simulink model "traiettoria_corretta (3)"  (R2022b)
settings: Solver=FixedStepAuto  StartTime=0.0  StopTime=70  RelTol=1e-3  EnableMultiTasking=on
PreLoadFcn:
  | if ispc
  | SampleTime = 0.01
  | PID_x_P = 8
  | PID_x_I = 0.1
  | PID_x_D = 10
  | PID_x_N = 10
  | 
  | PID_y_P = 8
  | PID_y_I = 0.1
  | PID_y_D = 6
  | PID_y_N = 10
  | 
  | PID_z_P = 1.13
  | PID_z_I = 0.1
  | PID_z_D = 0.8
  | PID_z_N = 100
  | 
  | PID_yaw_P = 0.08024000000000001
  | PID_yaw_I = 0.005
  | PID_yaw_D = 0.075
  | PID_yaw_N = 100
  | 
  | elseif isunix
  | SampleTime = 0.004
  | PID_x_P = 1
  | PID_x_I = 0.01
  | PID_x_D = 4
  | PID_x_N = 1
  | 
  | PID_y_P = 1
  | PID_y_I = 0.01
  | PID_y_D = 4
  | PID_y_N = 1
  | 
  | PID_z_P = 1
  | PID_z_I = 0.01
  | PID_z_D = 0.8
  | PID_z_N = 50
  | 
  | PID_yaw_P = 0.08024000000000001
  | PID_yaw_I = 0.005
  | PID_yaw_D = 0.075
  | PID_yaw_N = 100
  | end
undefined symbols (not defined in the file): dev, Main, pwm_output0
libraries: px4uORBlib x7, slpidlib x6, simulink_extras x3, px4Sensorslib x2, sharedtransform x1, SignalEditorBlockLib x1, px4lib x1
CloseFcn:
  | clear PID_yaw*;
  | clear PID_x*;
  | clear PID_y*;
  | clear PID_z*;
  | clear SampleTime;
settings Model: SimulationMode=external  ExtModeTrigDuration=3001  Creator=The MathWorks, Inc.  LastModifiedBy=utente
settings SolverCC: AlgebraicLoopSolver=TrustRegion  PositivePriorityOrder=on  AutoInsertRateTranBlk=on  MaxZcPerStep=1
settings OptimizationCC: EnhancedBackFolding=on  PassReuseOutputArgsAs=Individual arguments  ZeroExternalMemoryAtStartup=off  ZeroInternalMemoryAtStartup=off  MaxStackSize=64  OptimizeBlockOrder=speed  DifferentSizesBufferReuse=on  OptimizationCustomize=off  EfficientTunableParamExpr=on
settings DebuggingCC: MultiTaskDSMMsg=none  ParameterTunabilityLossMsg=error  UnconnectedInputMsg=warning  UnconnectedOutputMsg=warning  UnconnectedLineMsg=warning  SFMachineParentedDataDiag=warning
settings HardwareCC: ProdBitPerPointer=32  ProdBitPerSizeT=32  ProdBitPerPtrDiffT=32  ProdLargestAtomicInteger=Long  ProdLargestAtomicFloat=Double  ProdWordSize=32  ProdLongLongMode=on  ProdHWDeviceType=ARM Compatible->ARM Cortex
settings ModelReferenceCC: EnableRefExpFcnMdlSchedulingChecks=on
settings SFSimCC: MATLABDynamicMemAlloc=off  SimTargetLang=C++
settings RTWCC: Description=Embedded Coder  SystemTargetFile=ert.tlc  HardwareBoard=PX4 Host Target  TemplateMakefile=ert_default_tmf  Toolchain=GNU Tools for PX4 Autopilots  PortableWordSizes=on  TargetLang=C++  DLArmComputeVersion=19.05
settings CodeAppCC: ForceParamTrailComments=on  IgnoreCustomStorageClasses=off  OperatorAnnotations=on  SimulinkDataObjDesc=on  SFDataObjDesc=on  InsertBlockDesc=on
settings ERTTargetCC: ExtMode=on  ExtModeTransport=2  ExtModeStaticAlloc=on  ExtModeMexFile=ext_xcp  ExtModeMexArgs='127.0.0.1' 1 17725  ExtModeIntrfLevel=Level2 - Open

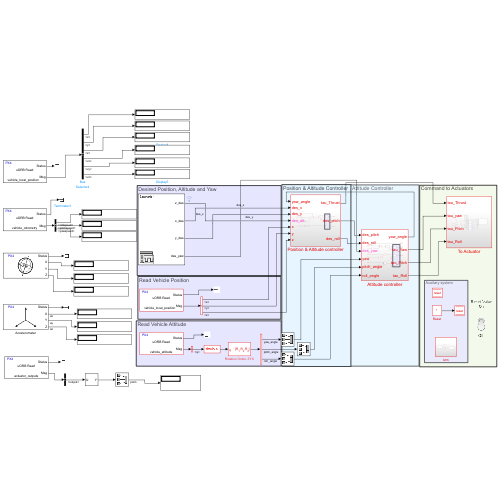
[thumbnail: Simulink's stored preview of the top-level diagram]
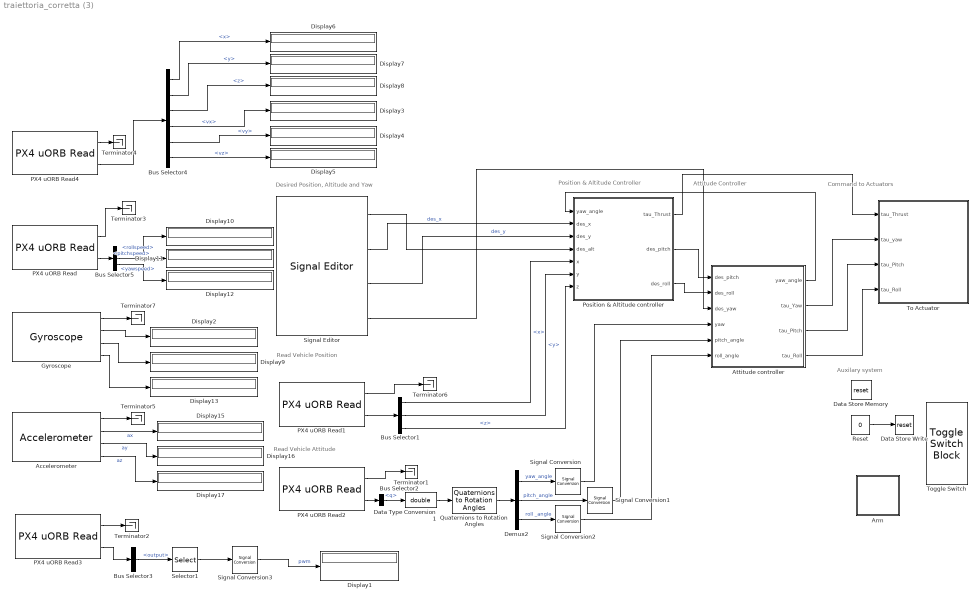
== system traiettoria_corretta (3) ==
  note: Read Vehicle Attitude
  note: Position & Altitude Controller
  note: Command to Actuators
  note: Auxilary system
  note: Attitude Controller
  note: Desired Position, Altitude and Yaw
  note: Read Vehicle Position
  Accelerometer : px4Sensorslib/Accelerometer  uorbTimeStamp=off  BlockingMode=off  BlockTimeout=1e-3  sampleTime=0.01
  Arm : Subsystem
  Attitude controller : Subsystem
  Bus Selector1 : BusSelector  OutputSignals=x,y,z
  Bus Selector2 : BusSelector  OutputSignals=q
  Bus Selector3 : BusSelector  OutputSignals=output
  Bus Selector4 : BusSelector  OutputSignals=x,y,z,vx,vy,vz
  Bus Selector5 : BusSelector  OutputSignals=rollspeed,pitchspeed,yawspeed
  Data Store Write : DataStoreWrite  DataStoreName=reset  IndexOptions=Index vector (dialog)  Indices=1  OutputSizes=1
  Data Store Memory : DataStoreMemory  DataStoreName=reset  ReadBeforeWriteMsg=warning  WriteAfterWriteMsg=warning  WriteAfterReadMsg=warning  ShowAdditionalParam=off  OutDataTypeStr=boolean
  Data Type Conversion1 : DataTypeConversion  OutDataTypeStr=double  SaturateOnIntegerOverflow=off  RndMeth=Floor
  Demux2 : Demux  Outputs=3
  Display{1..13,15..17} (16 alike) : Display
  Gyroscope : px4Sensorslib/Gyroscope  uorbTimeStamp=off  BlockingMode=off  BlockTimeout=1e-3  sampleTime=1/250
  PX4 uORB Read : px4uORBlib/PX4 uORB Read  uORBTopic=vehicle_odometry  selectInstance=vehicle_odometry  SampleTime=0.01  BlockingMode=off  BlockTimeout=1e-3
  PX4 uORB Read1 : px4uORBlib/PX4 uORB Read  uORBTopic=vehicle_local_position  selectInstance=vehicle_local_position_groundtruth  SampleTime=0.01  BlockingMode=off  BlockTimeout=1e-3
  PX4 uORB Read2 : px4uORBlib/PX4 uORB Read  uORBTopic=vehicle_attitude  selectInstance=vehicle_attitude_groundtruth  SampleTime=0.01  BlockingMode=off  BlockTimeout=1e-3
  PX4 uORB Read3 : px4uORBlib/PX4 uORB Read  uORBTopic=actuator_outputs  selectInstance=actuator_outputs  SampleTime=0.01  BlockingMode=off  BlockTimeout=1e-3
  PX4 uORB Read4 : px4uORBlib/PX4 uORB Read  uORBTopic=vehicle_local_position  selectInstance=vehicle_local_position_groundtruth  SampleTime=0.01  BlockingMode=off  BlockTimeout=1e-3
  Position & Altitude controller : Subsystem
  Quaternions to Rotation Angles : sharedtransform/Quaternions to Rotation Angles  rotationOrder=ZYX  aMode=aMode
  Reset : Constant  Value=0  OutDataTypeStr=boolean  SampleTime=-1
      settings: OpenFcn=|
      | if strcmp('0',get_param(gcb, 'Value'))                        set_param(gcb, 'Value', '1');
      | else
      |             set_param(gcb, 'Value', '0');
      | end
  Selector1 : Selector  InputPortWidth=16  IndexOptions=Index vector (dialog)  Indices=[1 2]  OutputSizes=1
  Signal Conversion{,1..3} (4 alike) : SignalConversion  OverrideOpt=off
  Signal Editor : SignalEditorBlockLib/Signal Editor  FileName=traiettoria_signal.mat  ActiveScenario=Scenario1  ActiveSignal=des_yaw  IsBus=off  OutputBusObjectStr=Bus: BusObject  SampleTime=0.01  Interpolate=off  ZeroCross=off  OutputAfterFinalValue=Setting to zero  Unit=inherit  PreserveSignalName=on
  Terminator{1..7} (7 alike) : Terminator
  To Actuator : Subsystem
  Toggle Switch : ToggleSwitchBlock
      settings: Values={{'Off', 'On'}, [0 1]}
  wires:
  Signal Editor/4 -> Attitude controller/3(des_yaw)
  Signal Editor/2 -> Position & Altitude controller/2(des_x)  "des_x"
  Bus Selector1/1 -> Position & Altitude controller/5(x)  "<x>"
  Bus Selector1/3 -> Position & Altitude controller/7(z)  "<z>"
  Position & Altitude controller/2(des_pitch) -> Attitude controller/1(des_pitch)
  Signal Editor/3 -> Position & Altitude controller/3(des_y)  "des_y"
  Demux2/1 -> Signal Conversion/1  "yaw_angle"
  Position & Altitude controller/1(tau_Thrust) -> To Actuator/1(tau_Thrust)
  Bus Selector2/1 -> Data Type Conversion1/1  "<q>"
  Data Type Conversion1/1 -> Quaternions to Rotation Angles/1
  Demux2/2 -> Signal Conversion1/1  "pitch_angle"
  PX4 uORB Read2/2 -> Bus Selector2/1
  PX4 uORB Read1/1 -> Terminator6/1
  PX4 uORB Read1/2 -> Bus Selector1/1
  Quaternions to Rotation Angles/1 -> Demux2/1
  Signal Editor/1 -> Position & Altitude controller/4(des_alt)
  Reset/1 -> Data Store Write/1
  Signal Conversion1/1 -> Attitude controller/5(pitch_angle)
  Bus Selector1/2 -> Position & Altitude controller/6(y)  "<y>"
  PX4 uORB Read2/1 -> Terminator1/1
  Attitude controller/2(tau_Yaw) -> To Actuator/2(tau_yaw)
  Attitude controller/3(tau_Pitch) -> To Actuator/3(tau_Pitch)
  Attitude controller/4(tau_Roll) -> To Actuator/4(tau_Roll)
  Attitude controller/1(yaw_angle) -> Position & Altitude controller/1(yaw_angle)
  Signal Conversion/1 -> Attitude controller/4(yaw)
  Signal Conversion2/1 -> Attitude controller/6(roll_angle)
  Position & Altitude controller/3(des_roll) -> Attitude controller/2(des_roll)
  Demux2/3 -> Signal Conversion2/1  "roll _angle"
  Gyroscope/1 -> Terminator7/1
  Gyroscope/2 -> Display2/1
  Gyroscope/3 -> Display9/1
  Gyroscope/4 -> Display13/1
  PX4 uORB Read3/1 -> Terminator2/1
  PX4 uORB Read3/2 -> Bus Selector3/1
  Bus Selector3/1 -> Selector1/1  "<output>"
  Selector1/1 -> Signal Conversion3/1
  Signal Conversion3/1 -> Display1/1  "pwm"
  PX4 uORB Read/1 -> Terminator3/1
  PX4 uORB Read/2 -> Bus Selector5/1
  Bus Selector5/1 -> Display10/1  "<rollspeed>"
  Bus Selector5/3 -> Display12/1  "<yawspeed>"
  Bus Selector5/2 -> Display11/1  "<pitchspeed>"
  PX4 uORB Read4/1 -> Terminator4/1
  PX4 uORB Read4/2 -> Bus Selector4/1
  Bus Selector4/1 -> Display6/1  "<x>"
  Bus Selector4/2 -> Display7/1  "<y>"
  Bus Selector4/3 -> Display8/1  "<z>"
  Bus Selector4/4 -> Display3/1  "<vx>"
  Bus Selector4/5 -> Display4/1  "<vy>"
  Bus Selector4/6 -> Display5/1  "<vz>"
  Accelerometer/1 -> Terminator5/1
  Accelerometer/2 -> Display15/1  "ax"
  Accelerometer/3 -> Display16/1  "ay"
  Accelerometer/4 -> Display17/1  "az"

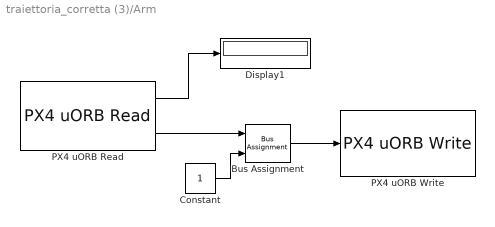
== system traiettoria_corretta (3)/Arm ==
  Bus Assignment : BusAssignment  AssignedSignals=armed
  Constant : Constant  OutDataTypeStr=Inherit: Inherit via back propagation  SampleTime=-1
  Display1 : Display
  PX4 uORB Read : px4uORBlib/PX4 uORB Read  uORBTopic=actuator_armed  selectInstance=actuator_armed  SampleTime=-1  BlockingMode=off  BlockTimeout=1e-3
  PX4 uORB Write : px4uORBlib/PX4 uORB Write  uORBTopic=actuator_armed  selectInstance=actuator_armed  MessageQueueLen=1
  wires:
  PX4 uORB Read/2 -> Bus Assignment/1
  PX4 uORB Read/1 -> Display1/1
  Bus Assignment/1 -> PX4 uORB Write/1
  Constant/1 -> Bus Assignment/2

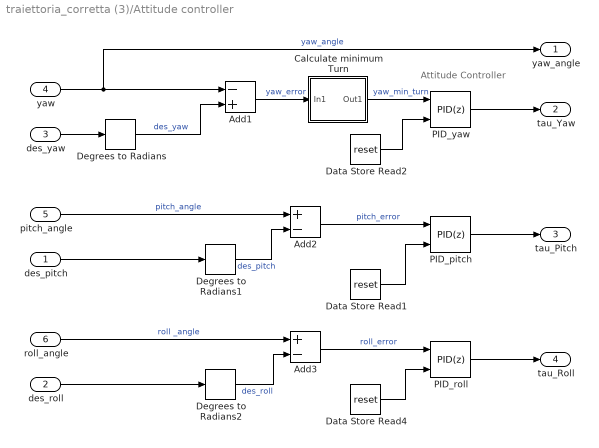
== system traiettoria_corretta (3)/Attitude controller ==
  note: Attitude Controller
  des_pitch : Inport
  des_roll : Inport  Port=2
  des_yaw : Inport  Port=3
  yaw : Inport  Port=4
  pitch_angle : Inport  Port=5
  roll_angle : Inport  Port=6
  Add1 : Sum  Inputs=-+
  Add2 : Sum  Inputs=+-
  Add3 : Sum  Inputs=+-
  Calculate minimum Turn : Subsystem
  Data Store Read1 : DataStoreRead  DataStoreName=reset  IndexOptions=Index vector (dialog)  Indices=1  OutputSizes=1
  Data Store Read2 : DataStoreRead  DataStoreName=reset  IndexOptions=Index vector (dialog)  Indices=1  OutputSizes=1
  Data Store Read4 : DataStoreRead  DataStoreName=reset  IndexOptions=Index vector (dialog)  Indices=1  OutputSizes=1
  Degrees to Radians : simulink_extras/Transformations/Degrees to Radians
  Degrees to Radians1 : simulink_extras/Transformations/Degrees to Radians
  Degrees to Radians2 : simulink_extras/Transformations/Degrees to Radians
  PID_pitch : slpidlib/PID Controller  Controller=PID  Form=Parallel  TimeDomain=Discrete-time  UseExternalTs=off  SampleTime=-1  IntegratorMethod=Backward Euler  FilterMethod=Forward Euler  ControllerParametersSource=internal  P=0.027  I=0.005  UseKiTs=off  D=0.0145948093220339  N=100  UseFilter=on  TunerSelectOption=Transfer Function Based (PID Tuner App)  InitialConditionSource=internal  InitialConditionForIntegrator=0  InitialConditionForFilter=0  DifferentiatorICPrevScaledInput=0  ExternalReset=level  TrackingMode=off  Kt=1  LimitOutput=on  SatLimitsSource=internal  UpperSaturationLimit=0.05  LowerSaturationLimit=-0.05  LinearizeAsGain=off  AntiWindupMode=none  Kb=1  LimitIntegrator=off  UpperIntegratorSaturationLimit=inf  LowerIntegratorSaturationLimit=-inf  POutMin=[]  POutMax=[]  IOutMin=[]  IOutMax=[]  DOutMin=[]  DOutMax=[]  NOutMin=[]  NOutMax=[]  SumOutMin=[]  SumOutMax=[]  SaturationOutMin=[]  SaturationOutMax=[]  PParamMin=[]  PParamMax=[]  IParamMin=[]  IParamMax=[]  DParamMin=[]  DParamMax=[]  NParamMin=[]  NParamMax=[]  KbParamMin=[]  KbParamMax=[]  KtParamMin=[]  KtParamMax=[]  KbOutMin=[]  KbOutMax=[]  KtOutMin=[]  KtOutMax=[]  IntegratorOutMin=[]  IntegratorOutMax=[]  FilterOutMin=[]  FilterOutMax=[]  SumI1OutMin=[]  SumI1OutMax=[]  SumI2OutMin=[]  SumI2OutMax=[]  SumI3OutMin=[]  SumI3OutMax=[]  SumI4OutMin=[]  SumI4OutMax=[]  SumDOutMin=[]  SumDOutMax=[]  DifferentiatorOutMin=[]  DifferentiatorOutMax=[]  FilterDiffOutCoefMin=[]  FilterDiffOutCoefMax=[]  ReciprocalOutMin=[]  ReciprocalOutMax=[]  SumDenOutMin=[]  SumDenOutMax=[]  SumNumOutMin=[]  SumNumOutMax=[]  DivideOutMin=[]  DivideOutMax=[]  UdiffTsProdOutMin=[]  UdiffTsProdOutMax=[]  NTsProdOutMin=[]  NTsProdOutMax=[]  UintegralTsProdOutMin=[]  UintegralTsProdOutMax=[]  UngainTsProdOutMin=[]  UngainTsProdOutMax=[]  ClampingZeroOutDataTypeStr=Inherit: Inherit via back propagation  ClampingZeroOutMin=[]  ClampingZeroOutMax=[]  FilterDenConstantOutDataTypeStr=Inherit: Inherit via back propagation  FilterDenConstantOutMin=[]  FilterDenConstantOutMax=[]  PCopyOutDataTypeStr=Inherit: Inherit via back propagation  PCopyOutMin=[]  PCopyOutMax=[]  NCopyOutDataTypeStr=Inherit: Inherit via back propagation  NCopyOutMin=[]  NCopyOutMax=[]  IntegratorContinuousStateAttributes=''  IntegratorStateMustResolveToSignalObject=off  IntegratorRTWStateStorageClass=Auto  FilterContinuousStateAttributes=''  FilterStateMustResolveToSignalObject=off  FilterRTWStateStorageClass=Auto  ParallelPVariant=InternalParameters  IdealPVariant=Disabled  IVariant=InternalParameters  DVariant=InternalParameters  IntegratorVariant=Discrete  SatVariant=Enabled  AWVariant=Passthrough  PCopyVariant=Disabled  TRVariant=Disabled  FdbkBlocksVariant=Forward  IdealPFdbkVariant=Disabled  SatFdbkVariant=Disabled  DerivativeFilterVariant=ForwardEulerFilter  NVariant=InternalParameters  NCopyVariant=Disabled  FilterICVariant=InternalICsFilter  IntegratorICVariant=InternalICs  ExternalResetVariant=ExternalReset  TRSumVariant=Passthrough  SumFdbkVariant=Disabled  SumVariant=Sum_PID  TsampFilterVariant=InternalTs  TsampNgainVariant=Passthrough  TsampIntegralVariant=Passthrough  ExternalSaturationOutDataTypeStr=Inherit: Same as second input
  PID_roll : slpidlib/PID Controller  Controller=PID  Form=Parallel  TimeDomain=Discrete-time  UseExternalTs=off  SampleTime=-1  IntegratorMethod=Backward Euler  FilterMethod=Forward Euler  ControllerParametersSource=internal  P=0.03  I=0.005  UseKiTs=off  D=0.015  N=100  UseFilter=on  TunerSelectOption=Transfer Function Based (PID Tuner App)  InitialConditionSource=internal  InitialConditionForIntegrator=0  InitialConditionForFilter=0  DifferentiatorICPrevScaledInput=0  ExternalReset=level  TrackingMode=off  Kt=1  LimitOutput=on  SatLimitsSource=internal  UpperSaturationLimit=0.05  LowerSaturationLimit=-0.05  LinearizeAsGain=off  AntiWindupMode=none  Kb=1  LimitIntegrator=off  UpperIntegratorSaturationLimit=inf  LowerIntegratorSaturationLimit=-inf  POutMin=[]  POutMax=[]  IOutMin=[]  IOutMax=[]  DOutMin=[]  DOutMax=[]  NOutMin=[]  NOutMax=[]  SumOutMin=[]  SumOutMax=[]  SaturationOutMin=[]  SaturationOutMax=[]  PParamMin=[]  PParamMax=[]  IParamMin=[]  IParamMax=[]  DParamMin=[]  DParamMax=[]  NParamMin=[]  NParamMax=[]  KbParamMin=[]  KbParamMax=[]  KtParamMin=[]  KtParamMax=[]  KbOutMin=[]  KbOutMax=[]  KtOutMin=[]  KtOutMax=[]  IntegratorOutMin=[]  IntegratorOutMax=[]  FilterOutMin=[]  FilterOutMax=[]  SumI1OutMin=[]  SumI1OutMax=[]  SumI2OutMin=[]  SumI2OutMax=[]  SumI3OutMin=[]  SumI3OutMax=[]  SumI4OutMin=[]  SumI4OutMax=[]  SumDOutMin=[]  SumDOutMax=[]  DifferentiatorOutMin=[]  DifferentiatorOutMax=[]  FilterDiffOutCoefMin=[]  FilterDiffOutCoefMax=[]  ReciprocalOutMin=[]  ReciprocalOutMax=[]  SumDenOutMin=[]  SumDenOutMax=[]  SumNumOutMin=[]  SumNumOutMax=[]  DivideOutMin=[]  DivideOutMax=[]  UdiffTsProdOutMin=[]  UdiffTsProdOutMax=[]  NTsProdOutMin=[]  NTsProdOutMax=[]  UintegralTsProdOutMin=[]  UintegralTsProdOutMax=[]  UngainTsProdOutMin=[]  UngainTsProdOutMax=[]  ClampingZeroOutDataTypeStr=Inherit: Inherit via back propagation  ClampingZeroOutMin=[]  ClampingZeroOutMax=[]  FilterDenConstantOutDataTypeStr=Inherit: Inherit via back propagation  FilterDenConstantOutMin=[]  FilterDenConstantOutMax=[]  PCopyOutDataTypeStr=Inherit: Inherit via back propagation  PCopyOutMin=[]  PCopyOutMax=[]  NCopyOutDataTypeStr=Inherit: Inherit via back propagation  NCopyOutMin=[]  NCopyOutMax=[]  IntegratorContinuousStateAttributes=''  IntegratorStateMustResolveToSignalObject=off  IntegratorRTWStateStorageClass=Auto  FilterContinuousStateAttributes=''  FilterStateMustResolveToSignalObject=off  FilterRTWStateStorageClass=Auto  ParallelPVariant=InternalParameters  IdealPVariant=Disabled  IVariant=InternalParameters  DVariant=InternalParameters  IntegratorVariant=Discrete  SatVariant=Enabled  AWVariant=Passthrough  PCopyVariant=Disabled  TRVariant=Disabled  FdbkBlocksVariant=Forward  IdealPFdbkVariant=Disabled  SatFdbkVariant=Disabled  DerivativeFilterVariant=ForwardEulerFilter  NVariant=InternalParameters  NCopyVariant=Disabled  FilterICVariant=InternalICsFilter  IntegratorICVariant=InternalICs  ExternalResetVariant=ExternalReset  TRSumVariant=Passthrough  SumFdbkVariant=Disabled  SumVariant=Sum_PID  TsampFilterVariant=InternalTs  TsampNgainVariant=Passthrough  TsampIntegralVariant=Passthrough  ExternalSaturationOutDataTypeStr=Inherit: Same as second input
  PID_yaw : slpidlib/PID Controller  Controller=PID  Form=Parallel  TimeDomain=Discrete-time  UseExternalTs=off  SampleTime=-1  IntegratorMethod=Backward Euler  FilterMethod=Forward Euler  ControllerParametersSource=internal  P=0.0802  I=0.0050  UseKiTs=off  D=0.0750  N=100  UseFilter=on  TunerSelectOption=Transfer Function Based (PID Tuner App)  InitialConditionSource=internal  InitialConditionForIntegrator=0  InitialConditionForFilter=0  DifferentiatorICPrevScaledInput=0  ExternalReset=level  TrackingMode=off  Kt=1  LimitOutput=on  SatLimitsSource=internal  UpperSaturationLimit=0.1  LowerSaturationLimit=-0.1  LinearizeAsGain=off  AntiWindupMode=none  Kb=1  LimitIntegrator=off  UpperIntegratorSaturationLimit=inf  LowerIntegratorSaturationLimit=-inf  POutMin=[]  POutMax=[]  IOutMin=[]  IOutMax=[]  DOutMin=[]  DOutMax=[]  NOutMin=[]  NOutMax=[]  SumOutMin=[]  SumOutMax=[]  SaturationOutMin=[]  SaturationOutMax=[]  PParamMin=[]  PParamMax=[]  IParamMin=[]  IParamMax=[]  DParamMin=[]  DParamMax=[]  NParamMin=[]  NParamMax=[]  KbParamMin=[]  KbParamMax=[]  KtParamMin=[]  KtParamMax=[]  KbOutMin=[]  KbOutMax=[]  KtOutMin=[]  KtOutMax=[]  IntegratorOutMin=[]  IntegratorOutMax=[]  FilterOutMin=[]  FilterOutMax=[]  SumI1OutMin=[]  SumI1OutMax=[]  SumI2OutMin=[]  SumI2OutMax=[]  SumI3OutMin=[]  SumI3OutMax=[]  SumI4OutMin=[]  SumI4OutMax=[]  SumDOutMin=[]  SumDOutMax=[]  DifferentiatorOutMin=[]  DifferentiatorOutMax=[]  FilterDiffOutCoefMin=[]  FilterDiffOutCoefMax=[]  ReciprocalOutMin=[]  ReciprocalOutMax=[]  SumDenOutMin=[]  SumDenOutMax=[]  SumNumOutMin=[]  SumNumOutMax=[]  DivideOutMin=[]  DivideOutMax=[]  UdiffTsProdOutMin=[]  UdiffTsProdOutMax=[]  NTsProdOutMin=[]  NTsProdOutMax=[]  UintegralTsProdOutMin=[]  UintegralTsProdOutMax=[]  UngainTsProdOutMin=[]  UngainTsProdOutMax=[]  ClampingZeroOutDataTypeStr=Inherit: Inherit via back propagation  ClampingZeroOutMin=[]  ClampingZeroOutMax=[]  FilterDenConstantOutDataTypeStr=Inherit: Inherit via back propagation  FilterDenConstantOutMin=[]  FilterDenConstantOutMax=[]  PCopyOutDataTypeStr=Inherit: Inherit via back propagation  PCopyOutMin=[]  PCopyOutMax=[]  NCopyOutDataTypeStr=Inherit: Inherit via back propagation  NCopyOutMin=[]  NCopyOutMax=[]  IntegratorContinuousStateAttributes=''  IntegratorStateMustResolveToSignalObject=off  IntegratorRTWStateStorageClass=Auto  FilterContinuousStateAttributes=''  FilterStateMustResolveToSignalObject=off  FilterRTWStateStorageClass=Auto  ParallelPVariant=InternalParameters  IdealPVariant=Disabled  IVariant=InternalParameters  DVariant=InternalParameters  IntegratorVariant=Discrete  SatVariant=Enabled  AWVariant=Passthrough  PCopyVariant=Disabled  TRVariant=Disabled  FdbkBlocksVariant=Forward  IdealPFdbkVariant=Disabled  SatFdbkVariant=Disabled  DerivativeFilterVariant=ForwardEulerFilter  NVariant=InternalParameters  NCopyVariant=Disabled  FilterICVariant=InternalICsFilter  IntegratorICVariant=InternalICs  ExternalResetVariant=ExternalReset  TRSumVariant=Passthrough  SumFdbkVariant=Disabled  SumVariant=Sum_PID  TsampFilterVariant=InternalTs  TsampNgainVariant=Passthrough  TsampIntegralVariant=Passthrough  ExternalSaturationOutDataTypeStr=Inherit: Same as second input
  yaw_angle : Outport
  tau_Yaw : Outport  Port=2
  tau_Pitch : Outport  Port=3
  tau_Roll : Outport  Port=4
  wires:
  des_pitch/1 -> Degrees to Radians1/1
  Degrees to Radians2/1 -> Add3/2  "des_roll"
  pitch_angle/1 -> Add2/1  "pitch_angle"
  Degrees to Radians1/1 -> Add2/2  "des_pitch"
  Add3/1 -> PID_roll/1  "roll_error"
  PID_yaw/1 -> tau_Yaw/1
  roll_angle/1 -> Add3/1  "roll _angle"
  des_yaw/1 -> Degrees to Radians/1
  Data Store Read2/1 -> PID_yaw/2
  Degrees to Radians/1 -> Add1/2  "des_yaw"
  Data Store Read4/1 -> PID_roll/2
  Add1/1 -> Calculate minimum Turn/1(In1)  "yaw_error"
  Data Store Read1/1 -> PID_pitch/2
  Add2/1 -> PID_pitch/1  "pitch_error"
  PID_roll/1 -> tau_Roll/1
  des_roll/1 -> Degrees to Radians2/1
  PID_pitch/1 -> tau_Pitch/1
  yaw/1 -> Add1/1, yaw_angle/1  "yaw_angle"
  Calculate minimum Turn/1(Out1) -> PID_yaw/1  "yaw_min_turn"

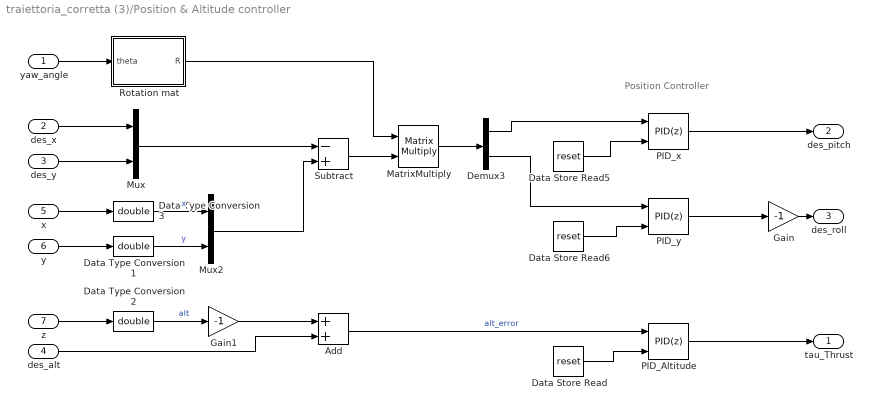
== system traiettoria_corretta (3)/Position & Altitude controller ==
  note: Position Controller
  yaw_angle : Inport
  des_x : Inport  Port=2
  des_y : Inport  Port=3
  des_alt : Inport  Port=4
  x : Inport  Port=5
  y : Inport  Port=6
  z : Inport  Port=7
  Add : Sum
  Data Store Read : DataStoreRead  DataStoreName=reset  IndexOptions=Index vector (dialog)  Indices=1  OutputSizes=1
  Data Store Read5 : DataStoreRead  DataStoreName=reset  IndexOptions=Index vector (dialog)  Indices=1  OutputSizes=1
  Data Store Read6 : DataStoreRead  DataStoreName=reset  IndexOptions=Index vector (dialog)  Indices=1  OutputSizes=1
  Data Type Conversion1 : DataTypeConversion  OutDataTypeStr=double  SaturateOnIntegerOverflow=off  RndMeth=Floor
  Data Type Conversion2 : DataTypeConversion  OutDataTypeStr=double  SaturateOnIntegerOverflow=off  RndMeth=Floor
  Data Type Conversion3 : DataTypeConversion  OutDataTypeStr=double  SaturateOnIntegerOverflow=off  RndMeth=Floor
  Demux3 : Demux  Outputs=2
  Gain : Gain  Gain=-1
  Gain1 : Gain  Gain=-1
  MatrixMultiply : Product  Multiplication=Matrix(*)
  Mux : Mux  Inputs=2
  Mux2 : Mux  Inputs=2
  PID_Altitude : slpidlib/PID Controller  Controller=PID  Form=Parallel  TimeDomain=Discrete-time  UseExternalTs=off  SampleTime=-1  IntegratorMethod=Backward Euler  FilterMethod=Forward Euler  ControllerParametersSource=internal  P=1  I=0.1  UseKiTs=off  D=0.8  N=100  UseFilter=on  TunerSelectOption=Transfer Function Based (PID Tuner App)  InitialConditionSource=internal  InitialConditionForIntegrator=1  InitialConditionForFilter=1  DifferentiatorICPrevScaledInput=0  ExternalReset=level  TrackingMode=off  Kt=1  LimitOutput=on  SatLimitsSource=internal  UpperSaturationLimit=2  LowerSaturationLimit=1  LinearizeAsGain=off  AntiWindupMode=clamping  Kb=1  LimitIntegrator=off  UpperIntegratorSaturationLimit=inf  LowerIntegratorSaturationLimit=-inf  POutMin=[]  POutMax=[]  IOutMin=[]  IOutMax=[]  DOutMin=[]  DOutMax=[]  NOutMin=[]  NOutMax=[]  SumOutMin=[]  SumOutMax=[]  SaturationOutMin=[]  SaturationOutMax=[]  PParamMin=[]  PParamMax=[]  IParamMin=[]  IParamMax=[]  DParamMin=[]  DParamMax=[]  NParamMin=[]  NParamMax=[]  KbParamMin=[]  KbParamMax=[]  KtParamMin=[]  KtParamMax=[]  KbOutMin=[]  KbOutMax=[]  KtOutMin=[]  KtOutMax=[]  IntegratorOutMin=[]  IntegratorOutMax=[]  FilterOutMin=[]  FilterOutMax=[]  SumI1OutMin=[]  SumI1OutMax=[]  SumI2OutMin=[]  SumI2OutMax=[]  SumI3OutMin=[]  SumI3OutMax=[]  SumI4OutMin=[]  SumI4OutMax=[]  SumDOutMin=[]  SumDOutMax=[]  DifferentiatorOutMin=[]  DifferentiatorOutMax=[]  FilterDiffOutCoefMin=[]  FilterDiffOutCoefMax=[]  ReciprocalOutMin=[]  ReciprocalOutMax=[]  SumDenOutMin=[]  SumDenOutMax=[]  SumNumOutMin=[]  SumNumOutMax=[]  DivideOutMin=[]  DivideOutMax=[]  UdiffTsProdOutMin=[]  UdiffTsProdOutMax=[]  NTsProdOutMin=[]  NTsProdOutMax=[]  UintegralTsProdOutMin=[]  UintegralTsProdOutMax=[]  UngainTsProdOutMin=[]  UngainTsProdOutMax=[]  ClampingZeroOutDataTypeStr=Inherit: Inherit via back propagation  ClampingZeroOutMin=[]  ClampingZeroOutMax=[]  FilterDenConstantOutDataTypeStr=Inherit: Inherit via back propagation  FilterDenConstantOutMin=[]  FilterDenConstantOutMax=[]  PCopyOutDataTypeStr=Inherit: Inherit via back propagation  PCopyOutMin=[]  PCopyOutMax=[]  NCopyOutDataTypeStr=Inherit: Inherit via back propagation  NCopyOutMin=[]  NCopyOutMax=[]  IntegratorContinuousStateAttributes=''  IntegratorStateMustResolveToSignalObject=off  IntegratorRTWStateStorageClass=Auto  FilterContinuousStateAttributes=''  FilterStateMustResolveToSignalObject=off  FilterRTWStateStorageClass=Auto  ParallelPVariant=InternalParameters  IdealPVariant=Disabled  IVariant=InternalParameters  DVariant=InternalParameters  IntegratorVariant=Discrete  SatVariant=Enabled  AWVariant=DiscClampingParallel  PCopyVariant=Disabled  TRVariant=Disabled  FdbkBlocksVariant=Feedback  IdealPFdbkVariant=Passthrough  SatFdbkVariant=Passthrough  DerivativeFilterVariant=ForwardEulerFilter  NVariant=InternalParameters  NCopyVariant=Disabled  FilterICVariant=InternalICsFilter  IntegratorICVariant=InternalICs  ExternalResetVariant=ExternalReset  TRSumVariant=Passthrough  SumFdbkVariant=Enabled  SumVariant=Sum_PID  TsampFilterVariant=InternalTs  TsampNgainVariant=Passthrough  TsampIntegralVariant=Passthrough  ExternalSaturationOutDataTypeStr=Inherit: Same as second input
  PID_x : slpidlib/PID Controller  Controller=PID  Form=Parallel  TimeDomain=Discrete-time  UseExternalTs=off  SampleTime=-1  IntegratorMethod=Forward Euler  FilterMethod=Forward Euler  ControllerParametersSource=internal  P=0.9  I=0.01  UseKiTs=off  D=3  N=1  UseFilter=on  TunerSelectOption=Transfer Function Based (PID Tuner App)  InitialConditionSource=internal  InitialConditionForIntegrator=0  InitialConditionForFilter=0  DifferentiatorICPrevScaledInput=0  ExternalReset=level  TrackingMode=off  Kt=1  LimitOutput=on  SatLimitsSource=internal  UpperSaturationLimit=50  LowerSaturationLimit=-50  LinearizeAsGain=off  AntiWindupMode=none  Kb=1  LimitIntegrator=off  UpperIntegratorSaturationLimit=inf  LowerIntegratorSaturationLimit=-inf  POutMin=[]  POutMax=[]  IOutMin=[]  IOutMax=[]  DOutMin=[]  DOutMax=[]  NOutMin=[]  NOutMax=[]  SumOutMin=[]  SumOutMax=[]  SaturationOutMin=[]  SaturationOutMax=[]  PParamMin=[]  PParamMax=[]  IParamMin=[]  IParamMax=[]  DParamMin=[]  DParamMax=[]  NParamMin=[]  NParamMax=[]  KbParamMin=[]  KbParamMax=[]  KtParamMin=[]  KtParamMax=[]  KbOutMin=[]  KbOutMax=[]  KtOutMin=[]  KtOutMax=[]  IntegratorOutMin=[]  IntegratorOutMax=[]  FilterOutMin=[]  FilterOutMax=[]  SumI1OutMin=[]  SumI1OutMax=[]  SumI2OutMin=[]  SumI2OutMax=[]  SumI3OutMin=[]  SumI3OutMax=[]  SumI4OutMin=[]  SumI4OutMax=[]  SumDOutMin=[]  SumDOutMax=[]  DifferentiatorOutMin=[]  DifferentiatorOutMax=[]  FilterDiffOutCoefMin=[]  FilterDiffOutCoefMax=[]  ReciprocalOutMin=[]  ReciprocalOutMax=[]  SumDenOutMin=[]  SumDenOutMax=[]  SumNumOutMin=[]  SumNumOutMax=[]  DivideOutMin=[]  DivideOutMax=[]  UdiffTsProdOutMin=[]  UdiffTsProdOutMax=[]  NTsProdOutMin=[]  NTsProdOutMax=[]  UintegralTsProdOutMin=[]  UintegralTsProdOutMax=[]  UngainTsProdOutMin=[]  UngainTsProdOutMax=[]  ClampingZeroOutDataTypeStr=Inherit: Inherit via back propagation  ClampingZeroOutMin=[]  ClampingZeroOutMax=[]  FilterDenConstantOutDataTypeStr=Inherit: Inherit via back propagation  FilterDenConstantOutMin=[]  FilterDenConstantOutMax=[]  PCopyOutDataTypeStr=Inherit: Inherit via back propagation  PCopyOutMin=[]  PCopyOutMax=[]  NCopyOutDataTypeStr=Inherit: Inherit via back propagation  NCopyOutMin=[]  NCopyOutMax=[]  IntegratorContinuousStateAttributes=''  IntegratorStateMustResolveToSignalObject=off  IntegratorRTWStateStorageClass=Auto  FilterContinuousStateAttributes=''  FilterStateMustResolveToSignalObject=off  FilterRTWStateStorageClass=Auto  ParallelPVariant=InternalParameters  IdealPVariant=Disabled  IVariant=InternalParameters  DVariant=InternalParameters  IntegratorVariant=Discrete  SatVariant=Enabled  AWVariant=Passthrough  PCopyVariant=Disabled  TRVariant=Disabled  FdbkBlocksVariant=Forward  IdealPFdbkVariant=Disabled  SatFdbkVariant=Disabled  DerivativeFilterVariant=ForwardEulerFilter  NVariant=InternalParameters  NCopyVariant=Disabled  FilterICVariant=InternalICsFilter  IntegratorICVariant=InternalICs  ExternalResetVariant=ExternalReset  TRSumVariant=Passthrough  SumFdbkVariant=Disabled  SumVariant=Sum_PID  TsampFilterVariant=InternalTs  TsampNgainVariant=Passthrough  TsampIntegralVariant=Passthrough  ExternalSaturationOutDataTypeStr=Inherit: Same as second input
  PID_y : slpidlib/PID Controller  Controller=PID  Form=Parallel  TimeDomain=Discrete-time  UseExternalTs=off  SampleTime=-1  IntegratorMethod=Forward Euler  FilterMethod=Forward Euler  ControllerParametersSource=internal  P=0.9  I=0.01  UseKiTs=off  D=3  N=1  UseFilter=on  TunerSelectOption=Transfer Function Based (PID Tuner App)  InitialConditionSource=internal  InitialConditionForIntegrator=0  InitialConditionForFilter=0  DifferentiatorICPrevScaledInput=0  ExternalReset=level  TrackingMode=off  Kt=1  LimitOutput=on  SatLimitsSource=internal  UpperSaturationLimit=50  LowerSaturationLimit=-50  LinearizeAsGain=off  AntiWindupMode=none  Kb=1  LimitIntegrator=off  UpperIntegratorSaturationLimit=inf  LowerIntegratorSaturationLimit=-inf  POutMin=[]  POutMax=[]  IOutMin=[]  IOutMax=[]  DOutMin=[]  DOutMax=[]  NOutMin=[]  NOutMax=[]  SumOutMin=[]  SumOutMax=[]  SaturationOutMin=[]  SaturationOutMax=[]  PParamMin=[]  PParamMax=[]  IParamMin=[]  IParamMax=[]  DParamMin=[]  DParamMax=[]  NParamMin=[]  NParamMax=[]  KbParamMin=[]  KbParamMax=[]  KtParamMin=[]  KtParamMax=[]  KbOutMin=[]  KbOutMax=[]  KtOutMin=[]  KtOutMax=[]  IntegratorOutMin=[]  IntegratorOutMax=[]  FilterOutMin=[]  FilterOutMax=[]  SumI1OutMin=[]  SumI1OutMax=[]  SumI2OutMin=[]  SumI2OutMax=[]  SumI3OutMin=[]  SumI3OutMax=[]  SumI4OutMin=[]  SumI4OutMax=[]  SumDOutMin=[]  SumDOutMax=[]  DifferentiatorOutMin=[]  DifferentiatorOutMax=[]  FilterDiffOutCoefMin=[]  FilterDiffOutCoefMax=[]  ReciprocalOutMin=[]  ReciprocalOutMax=[]  SumDenOutMin=[]  SumDenOutMax=[]  SumNumOutMin=[]  SumNumOutMax=[]  DivideOutMin=[]  DivideOutMax=[]  UdiffTsProdOutMin=[]  UdiffTsProdOutMax=[]  NTsProdOutMin=[]  NTsProdOutMax=[]  UintegralTsProdOutMin=[]  UintegralTsProdOutMax=[]  UngainTsProdOutMin=[]  UngainTsProdOutMax=[]  ClampingZeroOutDataTypeStr=Inherit: Inherit via back propagation  ClampingZeroOutMin=[]  ClampingZeroOutMax=[]  FilterDenConstantOutDataTypeStr=Inherit: Inherit via back propagation  FilterDenConstantOutMin=[]  FilterDenConstantOutMax=[]  PCopyOutDataTypeStr=Inherit: Inherit via back propagation  PCopyOutMin=[]  PCopyOutMax=[]  NCopyOutDataTypeStr=Inherit: Inherit via back propagation  NCopyOutMin=[]  NCopyOutMax=[]  IntegratorContinuousStateAttributes=''  IntegratorStateMustResolveToSignalObject=off  IntegratorRTWStateStorageClass=Auto  FilterContinuousStateAttributes=''  FilterStateMustResolveToSignalObject=off  FilterRTWStateStorageClass=Auto  ParallelPVariant=InternalParameters  IdealPVariant=Disabled  IVariant=InternalParameters  DVariant=InternalParameters  IntegratorVariant=Discrete  SatVariant=Enabled  AWVariant=Passthrough  PCopyVariant=Disabled  TRVariant=Disabled  FdbkBlocksVariant=Forward  IdealPFdbkVariant=Disabled  SatFdbkVariant=Disabled  DerivativeFilterVariant=ForwardEulerFilter  NVariant=InternalParameters  NCopyVariant=Disabled  FilterICVariant=InternalICsFilter  IntegratorICVariant=InternalICs  ExternalResetVariant=ExternalReset  TRSumVariant=Passthrough  SumFdbkVariant=Disabled  SumVariant=Sum_PID  TsampFilterVariant=InternalTs  TsampNgainVariant=Passthrough  TsampIntegralVariant=Passthrough  ExternalSaturationOutDataTypeStr=Inherit: Same as second input
  "Rotation mat " : MATLAB Function  TreatAsAtomicUnit=on
  Subtract : Sum  Inputs=-+
  tau_Thrust : Outport
  des_pitch : Outport  Port=2
  des_roll : Outport  Port=3
  wires:
  z/1 -> Data Type Conversion2/1
  "Rotation mat "/1(R) -> MatrixMultiply/1
  PID_Altitude/1 -> tau_Thrust/1
  Data Type Conversion3/1 -> Mux2/1  "x"
  Gain1/1 -> Add/1
  Mux/1 -> Subtract/1
  Demux3/1 -> PID_x/1
  des_x/1 -> Mux/1
  Data Type Conversion2/1 -> Gain1/1  "alt"
  MatrixMultiply/1 -> Demux3/1
  PID_x/1 -> des_pitch/1
  des_y/1 -> Mux/2
  Mux2/1 -> Subtract/2
  Data Store Read6/1 -> PID_y/2
  x/1 -> Data Type Conversion3/1
  des_alt/1 -> Add/2
  Data Store Read5/1 -> PID_x/2
  Data Type Conversion1/1 -> Mux2/2  "y"
  Subtract/1 -> MatrixMultiply/2
  Gain/1 -> des_roll/1
  y/1 -> Data Type Conversion1/1
  Add/1 -> PID_Altitude/1  "alt_error"
  yaw_angle/1 -> "Rotation mat "/1(theta)
  Demux3/2 -> PID_y/1
  Data Store Read/1 -> PID_Altitude/2
  PID_y/1 -> Gain/1

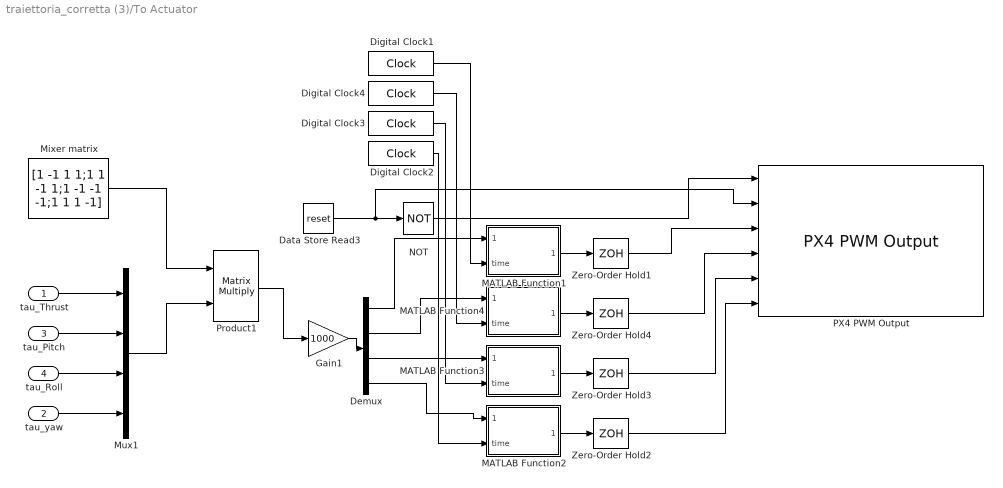
== system traiettoria_corretta (3)/To Actuator ==
  tau_Thrust : Inport
  tau_yaw : Inport  Port=2
  tau_Pitch : Inport  Port=3
  tau_Roll : Inport  Port=4
  Data Store Read3 : DataStoreRead  DataStoreName=reset  IndexOptions=Index vector (dialog)  Indices=1  OutputSizes=1
  Demux : Demux
  Digital Clock{1..4} (4 alike) : DigitalClock
  Gain1 : Gain  Gain=1000  OutDataTypeStr=uint16
  MATLAB Function1 : MATLAB Function  TreatAsAtomicUnit=on
  MATLAB Function2 : MATLAB Function  TreatAsAtomicUnit=on
  MATLAB Function3 : MATLAB Function  TreatAsAtomicUnit=on
  MATLAB Function4 : MATLAB Function  TreatAsAtomicUnit=on
  Mixer matrix : Constant  Value=[1 -1 1 1;1 1 -1 1;1 -1 -1 -1;1 1 1 -1]  OutDataTypeStr=Inherit: Inherit via back propagation
  Mux1 : Mux
  NOT : Logic  Operator=NOT  IconShape=distinctive  AllPortsSameDT=off  OutDataTypeStr=boolean
  PX4 PWM Output : px4lib/PX4 PWM Output  pwmDevice=Main (/dev/pwm_output0)  pwmChannel1_=on  pwmChannel2_=on  pwmChannel3_=on  pwmChannel4_=on  pwmChannel5_=off  pwmChannel6_=off  pwmChannel7_=off  pwmChannel8_=off  forceTerminateFailsafe=off  outputErrorStatus=off
  Product1 : Product  Multiplication=Matrix(*)  RndMeth=Zero
  Zero-Order Hold{1..4} (4 alike) : ZeroOrderHold  SampleTime=0.01
  wires:
  Product1/1 -> Gain1/1
  tau_Pitch/1 -> Mux1/2
  tau_Roll/1 -> Mux1/3
  Mux1/1 -> Product1/2
  tau_Thrust/1 -> Mux1/1
  Data Store Read3/1 -> PX4 PWM Output/2, NOT/1
  Gain1/1 -> Demux/1
  NOT/1 -> PX4 PWM Output/1
  tau_yaw/1 -> Mux1/4
  Mixer matrix/1 -> Product1/1
  Demux/1 -> MATLAB Function1/1(initialSpeed)
  Demux/4 -> MATLAB Function2/1(initialSpeed)
  Demux/2 -> MATLAB Function4/1(initialSpeed)
  Demux/3 -> MATLAB Function3/1(initialSpeed)
  Digital Clock1/1 -> MATLAB Function1/2(time)
  MATLAB Function1/1(deceleratedSpeed) -> Zero-Order Hold1/1
  Zero-Order Hold1/1 -> PX4 PWM Output/3
  Digital Clock2/1 -> MATLAB Function2/2(time)
  MATLAB Function2/1(deceleratedSpeed) -> Zero-Order Hold2/1
  Zero-Order Hold2/1 -> PX4 PWM Output/6
  Digital Clock3/1 -> MATLAB Function3/2(time)
  MATLAB Function3/1(deceleratedSpeed) -> Zero-Order Hold3/1
  Zero-Order Hold3/1 -> PX4 PWM Output/5
  Digital Clock4/1 -> MATLAB Function4/2(time)
  MATLAB Function4/1(deceleratedSpeed) -> Zero-Order Hold4/1
  Zero-Order Hold4/1 -> PX4 PWM Output/4

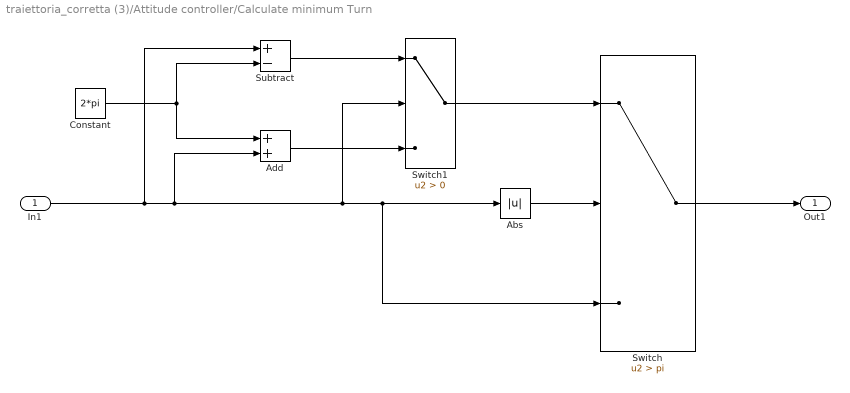
== system traiettoria_corretta (3)/Attitude controller/Calculate minimum Turn ==
  In1 : Inport
  Abs : Abs  SaturateOnIntegerOverflow=off
  Add : Sum
  Constant : Constant  Value=2*pi  SampleTime=-1
  Subtract : Sum  Inputs=+-
  Switch : Switch  Criteria=u2 > Threshold  Threshold=pi  SaturateOnIntegerOverflow=off  InputSameDT=off
  Switch1 : Switch  Criteria=u2 > Threshold  SaturateOnIntegerOverflow=off  InputSameDT=off
  Out1 : Outport
  wires:
  Switch/1 -> Out1/1
  Abs/1 -> Switch/2
  Constant/1 -> Subtract/2, Add/1
  Subtract/1 -> Switch1/1
  Add/1 -> Switch1/3
  In1/1 -> Subtract/1, Switch/3, Abs/1, Switch1/2, Add/2
  Switch1/1 -> Switch/1

== matlab function traiettoria_corretta (3)/To Actuator/MATLAB Function2 ==
  data: initialSpeed input; deceleratedSpeed output; time input
function deceleratedSpeed = decelerateSpeed(initialSpeed, time)
    persistent decelerationStarted;
    
    if isempty(decelerationStarted)
        decelerationStarted = false;
    end
    
   if time >= 38 && ~decelerationStarted
        decelerationStarted = true;
    end
    
    if decelerationStarted
        deceleratedSpeed = initialSpeed * exp(-0.08);
    else
        deceleratedSpeed = initialSpeed;
    end
end

== matlab function traiettoria_corretta (3)/To Actuator/MATLAB Function1 ==
  data: initialSpeed input; deceleratedSpeed output; time input
function deceleratedSpeed = decelerateSpeed(initialSpeed, time)
    persistent decelerationStarted;
    
    if isempty(decelerationStarted)
        decelerationStarted = false;
    end
    
   if time >= 35 && ~decelerationStarted
        decelerationStarted = true;
    end
    
    if decelerationStarted
        deceleratedSpeed = initialSpeed * exp(-0.05);
    else
        deceleratedSpeed = initialSpeed;
    end
end

== matlab function traiettoria_corretta (3)/To Actuator/MATLAB Function3 ==
  data: initialSpeed input; deceleratedSpeed output; time input
function deceleratedSpeed = decelerateSpeed(initialSpeed, time)
    persistent decelerationStarted;
    
    if isempty(decelerationStarted)
        decelerationStarted = false;
    end
    
   if time >= 37 && ~decelerationStarted
        decelerationStarted = true;
    end
    
    if decelerationStarted
        deceleratedSpeed = initialSpeed * exp(-0.08);
    else
        deceleratedSpeed = initialSpeed;
    end
end

== matlab function traiettoria_corretta (3)/To Actuator/MATLAB Function4 ==
  data: initialSpeed input; deceleratedSpeed output; time input
function deceleratedSpeed = decelerateSpeed(initialSpeed, time)
    persistent decelerationStarted;
    
    if isempty(decelerationStarted)
        decelerationStarted = false;
    end
    
   if time >= 36 && ~decelerationStarted
        decelerationStarted = true;
    end
    
    if decelerationStarted
        deceleratedSpeed = initialSpeed * exp(-0.08);
    else
        deceleratedSpeed = initialSpeed;
    end
end

== matlab function traiettoria_corretta (3)/Position & Altitude controller/Rotation mat  ==
  data: theta input; R output
function R = fcn(theta)
R = [cos(theta) -sin(theta); sin(theta) cos(theta)]';
